simulink model "Hector_Simulation"  (R2023b)
settings: Solver=daessc  StartTime=0.0  StopTime=8  FixedStep=0.001  MaxStep=1e-3  RelTol=1e-2
model workspace (MATLAB code in the model file):
  | %% World Plane
  | plane_x = 20;
  | plane_y = 2;
  | plane_z = 0.05;
  | 
  | %% motor
  | %A1
  | motor_com = [0, -0.02,0];
  | motor_com_mirror = [0, 0.02,0];
  | 
  | motor_I = [0.00048,0.00071,0.00048];
  | motor_mass = 0.605;
  | 
  | %% Body
  | % Inertial
  | body_com_x = 0.0;
  | body_com_y = 0.0;
  | body_com_z = -0.0;
  | body_mass = 5.75;
  | body_ixx = 44350*1e-6;
  | body_ixy = 0.0;
  | body_ixz = 0.0;
  | body_iyy = 53149*1e-6;
  | body_iyz = 0.0;
  | body_izz = 21390*1e-6;
  | 
  | %% Hip 1
  | % joint
  | hip1_offset_x =0.0;
  | hip1_offset_y = 0.047;
  | hip1_offset_z = 0.1265;
  | % hip1_max = 15;
  | % hip1_min = -15;
  | hip1_velocity_max = 21;
  | hip1_torque_max = 33.5;
  | % Inertial
  | hip1_com_x = 0.0268;
  | hip1_com_y = -0.00315;
  | hip1_com_z = -0.0272;
  | hip1_mass = 0.173;
  | hip1_ixx = 0.00022;
  | hip1_ixy = 0.0;
  | hip1_ixz = 0.0;
  | hip1_iyy = 0.00024;
  | hip1_iyz = 0.0;
  | hip1_izz = 0.00016;
  | 
  | %% Hip 2
  | % joint
  | hip2_offset_x =0.053;
  | hip2_offset_y = 0.0185;
  | hip2_offset_z = 0.071;
  | % hip2_max = 15;
  | % hip2_min = -15;
  | hip2_velocity_max = 21;
  | hip2_torque_max = 33.5;
  | % Inertial
  | hip2_com_x = -0.0308;
  | hip2_com_y = -0.00942;
  | hip2_com_z = 0.0;
  | hip2_mass = 0.0722;
  | hip2_ixx = 0.0000422;
  | hip2_ixy = 0.0;
  | hip2_ixz = 0.0;
  | hip2_iyy = 0.000120;
  | hip2_iyz = 0.0;
  | hip2_izz = 0.0000708;
  | 
  | %% Thigh
  | % joint
  | thigh_offset_x =-0.06;
  | thigh_offset_y = 0.004;
  | thigh_offset_z = 0.0;
  | % thigh_max = 130;
  | % thigh_min = -45;
  | thigh_velocity_max = 21;
  | thigh_torque_max = 33.5;
  | % Inertial
  | thigh_com_x = -0.00143;
  | thigh_com_y = -0.02106;
  | thigh_com_z = -0.06115;
  | thigh_mass = 0.397;
  | thigh_ixx = 0.00197;
  | thigh_ixy = 0.0;
  | thigh_ixz = 0.0;
  | thigh_iyy = 0.00218;
  | thigh_iyz = 0.0;
  | thigh_izz = 0.00033;
  | 
  | ankle_motor_offset_x = 0;
  | ankle_motor_offset_y = 0.039;
  | ankle_motor_offset_z = 0;
  | 
  | knee_motor_offset_x = 0;
  | knee_motor_offset_y = 0.039;
  | knee_motor_offset_z = -0.095;
  | 
  | %% Calf
  | % joint
  | calf_offset_x = 0.0;
  | calf_offset_y = 0.003;
  | calf_offset_z = -0.22;
  | % calf_max = 0;
  | % calf_min = -135;
  | % knee_max = 0;
  | % knee_min = -160;
  | calf_velocity_max = 14*1.5;
  | calf_torque_max = 51;
  | % Inertial
  | calf_com_x = 0.00165;
  | calf_com_y = -0.01117;
  | calf_com_z = -0.06438;
  | calf_mass = 0.136;
  | calf_ixx = 0.00071;
  | calf_ixy = 0.0;
  | calf_ixz = 0.0;
  | calf_iyy = 0.00072;
  | calf_iyz = 0.0;
  | calf_izz = 0.00002;
  | 
  | %% Toe
  | % joint
  | toe_offset_x = 0.0;
  | toe_offset_y = 0.011;
  | toe_offset_z = -0.22;
  | % toe_max = 60;
  | % toe_min = -60;
  | toe_velocity_max = 21;
  | toe_torque_max = 33.5;
  | % Inertial
  | toe_com_x = 0.00239;
  | toe_com_y = 0.00002;
  | toe_com_z = -0.02261;
  | toe_mass = 0.08425;
  | toe_ixx = 0.00001;
  | toe_ixy = 0.0;
  | toe_ixz = 0.0;
  | toe_iyy = 0.00011;
  | toe_iyz = 0.0;
  | toe_izz = 0.00011;
  | %% Contact
  | contact_front = 0.091;
  | contact_rear = -0.061;
  | contact_right = 0.026;
  | contact_left = 0.01;
  | contact_z = 0.039;
  | 
  | %%
  | %dorito
  | dorito_offset_x = 0;
  | dorito_offset_y = 0.012;
  | dorito_offset_z = 0;
  | 
  | dorito_lower_connection = [0.034 0 -0.044];
  | dorito_upper_connection = [0.034 0 0.021];
  | 
  | linkage_mass = 0.051;
  | linkage_com = [0 0 -0.11];
  | linkage_I = [0.00001 0.00002 0.00002];
  | %% Arms
  | shoulder_com_x = 0;
  | shoulder_com_y = 0;
  | shoulder_com_z = 0;
  | shoulder_mass = 0.835;
  | % shoulder_mass = 0.05;
  | shoulder_ixx = 920*1e-6;
  | shoulder_ixy = 0.0;
  | shoulder_ixz = 0.0;
  | shoulder_iyy = 270*1e-6;
  | shoulder_iyz = 0.0;
  | shoulder_izz = 499*1e-6;
  | 
  | upperarm_com_x = 0;
  | upperarm_com_y = 0;
  | upperarm_com_z = 0;
  | upperarm_mass = 1.35;
  | % upperarm_mass = 0.05;
  | upperarm_ixx = 1200*1e-6;
  | upperarm_ixy = 0.0;
  | upperarm_ixz = 0.0;
  | upperarm_iyy = 1170*1e-6;
  | upperarm_iyz = 0.0;
  | upperarm_izz = 729*1e-6;
  | 
  | forearm_com_x = 0;
  | forearm_com_y = 0;
  | forearm_com_z = -0.10;
  | forearm_mass = 0.53;
  | % forearm_mass = 0.03;
  | forearm_ixx = 427*1e-6;
  | forearm_ixy = 0.0;
  | forearm_ixz = 0.0;
  | forearm_iyy = 466*1e-6;
  | forearm_iyz = 0.0;
  | forearm_izz = 72*1e-6;
values from neighbouring files (symbols this model uses):
  body_v0 = [0 0 0]    [Initiate_Simulation.m]
  body_z0 = 0.55    [Initiate_Simulation.m]
  dt_MPC = gaitcycle/10    (= 0.04)    [Initiate_Simulation.m]
  map = rot90(z_heights) > 0    [Occupancy_Map.m]
  N = 5000    [Initiate_Simulation.m]
  q_goal = [4; 0; body_z0]    [Initiate_Simulation.m]    (also in artificialPotential.m = reshape(u(3:4), 2, 1); main.m = [20; 20])
  shoulderx_max = 90    [Initiate_Simulation.m]
  shoulderx_min = -15    [Initiate_Simulation.m]
  shoulderx_q0 = 0    [Initiate_Simulation.m]
undefined symbols (not defined in the file or in its folder): AssignMPCStage, sigbuilder_block, X, Y, Z
libraries: sm_lib x169, nesl_utility x95, dspindex x1, simulink x1
(part 6 of 7)

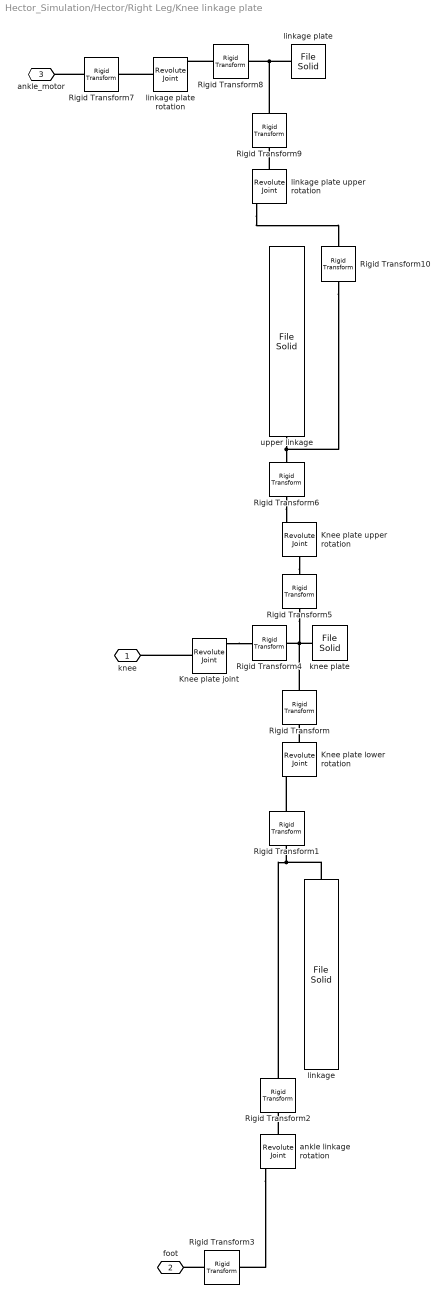
== system Hector_Simulation/Hector/Right Leg/Knee linkage plate ==
  Knee plate joint : sm_lib/Joints/Revolute Joint  JointMode=Normal  SenseConstraintForce=off  SenseConstraintForceX=off  SenseConstraintForceY=off  SenseConstraintForceZ=off  SenseConstraintTorque=off  SenseConstraintTorqueX=off  SenseConstraintTorqueY=off  SenseConstraintTorqueZ=off  SenseTotalForce=off  SenseTotalForceX=off  SenseTotalForceY=off  SenseTotalForceZ=off  SenseTotalTorque=off  SenseTotalTorqueX=off  SenseTotalTorqueY=off  SenseTotalTorqueZ=off  CompositeWrenchDir=FollowerOnBase  CompositeWrenchFrame=BaseFrame  EquilibriumPosition=0  EquilibriumPositionUnits=deg  SpringStiffness=0  SpringStiffnessUnits=N*m/deg  DampingCoefficient=joint_damping  DampingCoefficientUnits=N*m/(rad/s)  TorqueActuationMode=NoTorque  MotionActuationMode=ComputedMotion  SensePosition=on  SenseVelocity=on  SenseAcceleration=off  SenseTorqueForce=off  SenseLowerLimitTorqueForce=off  SenseUpperLimitTorqueForce=off  LowerLimitSpecify=off  LowerLimitBound=knee_min  LowerLimitBoundUnits=deg  LowerLimitStiffness=limit_stiffness  LowerLimitStiffnessUnits=N*m/deg  LowerLimitDamping=limit_damping  LowerLimitDampingUnits=N*m/(deg/s)  LowerLimitTransitionRegionWidth=0.1  LowerLimitTransitionRegionWidthUnits=deg  UpperLimitSpecify=off  UpperLimitBound=knee_max  UpperLimitBoundUnits=deg  UpperLimitStiffness=limit_stiffness  UpperLimitStiffnessUnits=N*m/deg  UpperLimitDamping=limit_damping  UpperLimitDampingUnits=N*m/(deg/s)  UpperLimitTransitionRegionWidth=0.1  UpperLimitTransitionRegionWidthUnits=deg  PositionTargetSpecify=off  PositionTargetPriority=High  PositionTargetValue=calf_q0  PositionTargetValueUnits=deg  VelocityTargetSpecify=off  VelocityTargetPriority=High  VelocityTargetValue=0  VelocityTargetValueUnits=deg/s
  Knee plate lower rotation : sm_lib/Joints/Revolute Joint  JointMode=Normal  SenseConstraintForce=off  SenseConstraintForceX=off  SenseConstraintForceY=off  SenseConstraintForceZ=off  SenseConstraintTorque=off  SenseConstraintTorqueX=off  SenseConstraintTorqueY=off  SenseConstraintTorqueZ=off  SenseTotalForce=off  SenseTotalForceX=off  SenseTotalForceY=off  SenseTotalForceZ=off  SenseTotalTorque=off  SenseTotalTorqueX=off  SenseTotalTorqueY=off  SenseTotalTorqueZ=off  CompositeWrenchDir=FollowerOnBase  CompositeWrenchFrame=BaseFrame  EquilibriumPosition=0  EquilibriumPositionUnits=deg  SpringStiffness=0  SpringStiffnessUnits=N*m/deg  DampingCoefficient=joint_damping  DampingCoefficientUnits=N*m/(rad/s)  TorqueActuationMode=NoTorque  MotionActuationMode=ComputedMotion  SensePosition=on  SenseVelocity=on  SenseAcceleration=off  SenseTorqueForce=off  SenseLowerLimitTorqueForce=off  SenseUpperLimitTorqueForce=off  LowerLimitSpecify=off  LowerLimitBound=knee_min  LowerLimitBoundUnits=deg  LowerLimitStiffness=limit_stiffness  LowerLimitStiffnessUnits=N*m/deg  LowerLimitDamping=limit_damping  LowerLimitDampingUnits=N*m/(deg/s)  LowerLimitTransitionRegionWidth=0.1  LowerLimitTransitionRegionWidthUnits=deg  UpperLimitSpecify=off  UpperLimitBound=knee_max  UpperLimitBoundUnits=deg  UpperLimitStiffness=limit_stiffness  UpperLimitStiffnessUnits=N*m/deg  UpperLimitDamping=limit_damping  UpperLimitDampingUnits=N*m/(deg/s)  UpperLimitTransitionRegionWidth=0.1  UpperLimitTransitionRegionWidthUnits=deg  PositionTargetSpecify=off  PositionTargetPriority=High  PositionTargetValue=calf_q0  PositionTargetValueUnits=deg  VelocityTargetSpecify=off  VelocityTargetPriority=High  VelocityTargetValue=0  VelocityTargetValueUnits=deg/s
  Knee plate upper rotation : sm_lib/Joints/Revolute Joint  JointMode=Normal  SenseConstraintForce=off  SenseConstraintForceX=off  SenseConstraintForceY=off  SenseConstraintForceZ=off  SenseConstraintTorque=off  SenseConstraintTorqueX=off  SenseConstraintTorqueY=off  SenseConstraintTorqueZ=off  SenseTotalForce=off  SenseTotalForceX=off  SenseTotalForceY=off  SenseTotalForceZ=off  SenseTotalTorque=off  SenseTotalTorqueX=off  SenseTotalTorqueY=off  SenseTotalTorqueZ=off  CompositeWrenchDir=FollowerOnBase  CompositeWrenchFrame=BaseFrame  EquilibriumPosition=0  EquilibriumPositionUnits=deg  SpringStiffness=0  SpringStiffnessUnits=N*m/deg  DampingCoefficient=joint_damping  DampingCoefficientUnits=N*m/(rad/s)  TorqueActuationMode=NoTorque  MotionActuationMode=ComputedMotion  SensePosition=on  SenseVelocity=on  SenseAcceleration=off  SenseTorqueForce=off  SenseLowerLimitTorqueForce=off  SenseUpperLimitTorqueForce=off  LowerLimitSpecify=off  LowerLimitBound=knee_min  LowerLimitBoundUnits=deg  LowerLimitStiffness=limit_stiffness  LowerLimitStiffnessUnits=N*m/deg  LowerLimitDamping=limit_damping  LowerLimitDampingUnits=N*m/(deg/s)  LowerLimitTransitionRegionWidth=0.1  LowerLimitTransitionRegionWidthUnits=deg  UpperLimitSpecify=off  UpperLimitBound=knee_max  UpperLimitBoundUnits=deg  UpperLimitStiffness=limit_stiffness  UpperLimitStiffnessUnits=N*m/deg  UpperLimitDamping=limit_damping  UpperLimitDampingUnits=N*m/(deg/s)  UpperLimitTransitionRegionWidth=0.1  UpperLimitTransitionRegionWidthUnits=deg  PositionTargetSpecify=off  PositionTargetPriority=High  PositionTargetValue=calf_q0  PositionTargetValueUnits=deg  VelocityTargetSpecify=off  VelocityTargetPriority=High  VelocityTargetValue=0  VelocityTargetValueUnits=deg/s
  Rigid Transform : sm_lib/Frames and Transforms/Rigid Transform  TranslationMethod=Cartesian  TranslationStandardOffset=0  TranslationStandardOffsetUnits=m  TranslationStandardAxis=+Z  TranslationCartesianOffset=dorito_lower_connection  TranslationCartesianOffsetUnits=m  TranslationROffset=0  TranslationROffsetUnits=m  TranslationZOffset=0  TranslationZOffsetUnits=m  TranslationThetaOffset=0  TranslationThetaOffsetUnits=deg  RotationMethod=StandardAxis  RotationAngleUnits=deg  RotationStandardAxis=+X  RotationAngle=90  RotationArbitraryAxis=[0 0 1]  FollAlignAxisA=+X  BaseAlignAxisA=+Y  FollAlignAxisB=+Y  BaseAlignAxisB=+Z  RotationSequenceAxes=FollowerAxes  RotationSequence=XYX  RotationSequenceAngles=[0 0 0]  RotationSequenceAnglesUnits=deg  RotationMatrix=[1 0 0; 0 1 0; 0 0 1]  Quaternion=[1 0 0 0]
  Rigid Transform1 : sm_lib/Frames and Transforms/Rigid Transform  TranslationMethod=None  TranslationStandardOffset=0  TranslationStandardOffsetUnits=m  TranslationStandardAxis=+Z  TranslationCartesianOffset=dorito_lower_connection  TranslationCartesianOffsetUnits=m  TranslationROffset=0  TranslationROffsetUnits=m  TranslationZOffset=0  TranslationZOffsetUnits=m  TranslationThetaOffset=0  TranslationThetaOffsetUnits=deg  RotationMethod=RotationSequence  RotationAngleUnits=deg  RotationStandardAxis=+X  RotationAngle=90  RotationArbitraryAxis=[0 0 1]  FollAlignAxisA=+X  BaseAlignAxisA=+Y  FollAlignAxisB=+Y  BaseAlignAxisB=+Z  RotationSequenceAxes=FollowerAxes  RotationSequence=XYZ  RotationSequenceAngles=[0 90 90]  RotationSequenceAnglesUnits=deg  RotationMatrix=[1 0 0; 0 1 0; 0 0 1]  Quaternion=[1 0 0 0]
  Rigid Transform10 : sm_lib/Frames and Transforms/Rigid Transform  TranslationMethod=Cartesian  TranslationStandardOffset=0  TranslationStandardOffsetUnits=m  TranslationStandardAxis=+Z  TranslationCartesianOffset=[0 0 -0.22]  TranslationCartesianOffsetUnits=m  TranslationROffset=0  TranslationROffsetUnits=m  TranslationZOffset=0  TranslationZOffsetUnits=m  TranslationThetaOffset=0  TranslationThetaOffsetUnits=deg  RotationMethod=StandardAxis  RotationAngleUnits=deg  RotationStandardAxis=-X  RotationAngle=90  RotationArbitraryAxis=[0 0 1]  FollAlignAxisA=+X  BaseAlignAxisA=+Y  FollAlignAxisB=+Y  BaseAlignAxisB=+Z  RotationSequenceAxes=FollowerAxes  RotationSequence=XYZ  RotationSequenceAngles=[0 90 90]  RotationSequenceAnglesUnits=deg  RotationMatrix=[1 0 0; 0 1 0; 0 0 1]  Quaternion=[1 0 0 0]
  Rigid Transform2 : sm_lib/Frames and Transforms/Rigid Transform  TranslationMethod=Cartesian  TranslationStandardOffset=0  TranslationStandardOffsetUnits=m  TranslationStandardAxis=+Z  TranslationCartesianOffset=[0 0 -0.22]  TranslationCartesianOffsetUnits=m  TranslationROffset=0  TranslationROffsetUnits=m  TranslationZOffset=0  TranslationZOffsetUnits=m  TranslationThetaOffset=0  TranslationThetaOffsetUnits=deg  RotationMethod=RotationSequence  RotationAngleUnits=deg  RotationStandardAxis=+X  RotationAngle=90  RotationArbitraryAxis=[0 0 1]  FollAlignAxisA=+X  BaseAlignAxisA=+Y  FollAlignAxisB=+Y  BaseAlignAxisB=+Z  RotationSequenceAxes=FollowerAxes  RotationSequence=XYZ  RotationSequenceAngles=[-90 0 0]  RotationSequenceAnglesUnits=deg  RotationMatrix=[1 0 0; 0 1 0; 0 0 1]  Quaternion=[1 0 0 0]
  Rigid Transform3 : sm_lib/Frames and Transforms/Rigid Transform  TranslationMethod=Cartesian  TranslationStandardOffset=0  TranslationStandardOffsetUnits=m  TranslationStandardAxis=+Z  TranslationCartesianOffset=[0.0475 -0.0275 0.001 ]  TranslationCartesianOffsetUnits=m  TranslationROffset=0  TranslationROffsetUnits=m  TranslationZOffset=0  TranslationZOffsetUnits=m  TranslationThetaOffset=0  TranslationThetaOffsetUnits=deg  RotationMethod=StandardAxis  RotationAngleUnits=deg  RotationStandardAxis=+X  RotationAngle=90  RotationArbitraryAxis=[0 0 1]  FollAlignAxisA=+X  BaseAlignAxisA=+Y  FollAlignAxisB=+Y  BaseAlignAxisB=+Z  RotationSequenceAxes=FollowerAxes  RotationSequence=XYZ  RotationSequenceAngles=[90 0 180]  RotationSequenceAnglesUnits=deg  RotationMatrix=[1 0 0; 0 1 0; 0 0 1]  Quaternion=[1 0 0 0]
  Rigid Transform4 : sm_lib/Frames and Transforms/Rigid Transform  TranslationMethod=Cartesian  TranslationStandardOffset=0  TranslationStandardOffsetUnits=m  TranslationStandardAxis=+Z  TranslationCartesianOffset=[dorito_offset_x -dorito_offset_y dorito_offset_z]  TranslationCartesianOffsetUnits=m  TranslationROffset=0  TranslationROffsetUnits=m  TranslationZOffset=0  TranslationZOffsetUnits=m  TranslationThetaOffset=0  TranslationThetaOffsetUnits=deg  RotationMethod=RotationSequence  RotationAngleUnits=deg  RotationStandardAxis=+Z  RotationAngle=90  RotationArbitraryAxis=[0 0 1]  FollAlignAxisA=+X  BaseAlignAxisA=+Y  FollAlignAxisB=+Y  BaseAlignAxisB=+Z  RotationSequenceAxes=FollowerAxes  RotationSequence=XYZ  RotationSequenceAngles=[90 0 180]  RotationSequenceAnglesUnits=deg  RotationMatrix=[1 0 0; 0 1 0; 0 0 1]  Quaternion=[1 0 0 0]
  Rigid Transform5 : sm_lib/Frames and Transforms/Rigid Transform  TranslationMethod=Cartesian  TranslationStandardOffset=0  TranslationStandardOffsetUnits=m  TranslationStandardAxis=+Z  TranslationCartesianOffset=[dorito_upper_connection(1), dorito_upper_connection(2), dorito_upper_connection(3)]  TranslationCartesianOffsetUnits=m  TranslationROffset=0  TranslationROffsetUnits=m  TranslationZOffset=0  TranslationZOffsetUnits=m  TranslationThetaOffset=0  TranslationThetaOffsetUnits=deg  RotationMethod=StandardAxis  RotationAngleUnits=deg  RotationStandardAxis=+X  RotationAngle=90  RotationArbitraryAxis=[0 0 1]  FollAlignAxisA=+X  BaseAlignAxisA=+Y  FollAlignAxisB=+Y  BaseAlignAxisB=+Z  RotationSequenceAxes=FollowerAxes  RotationSequence=XYX  RotationSequenceAngles=[0 0 0]  RotationSequenceAnglesUnits=deg  RotationMatrix=[1 0 0; 0 1 0; 0 0 1]  Quaternion=[1 0 0 0]
  Rigid Transform6 : sm_lib/Frames and Transforms/Rigid Transform  TranslationMethod=None  TranslationStandardOffset=0  TranslationStandardOffsetUnits=m  TranslationStandardAxis=+Z  TranslationCartesianOffset=dorito_lower_connection  TranslationCartesianOffsetUnits=m  TranslationROffset=0  TranslationROffsetUnits=m  TranslationZOffset=0  TranslationZOffsetUnits=m  TranslationThetaOffset=0  TranslationThetaOffsetUnits=deg  RotationMethod=RotationSequence  RotationAngleUnits=deg  RotationStandardAxis=+X  RotationAngle=90  RotationArbitraryAxis=[0 0 1]  FollAlignAxisA=+X  BaseAlignAxisA=+Y  FollAlignAxisB=+Y  BaseAlignAxisB=+Z  RotationSequenceAxes=FollowerAxes  RotationSequence=XYZ  RotationSequenceAngles=[0 90 90]  RotationSequenceAnglesUnits=deg  RotationMatrix=[1 0 0; 0 1 0; 0 0 1]  Quaternion=[1 0 0 0]
  Rigid Transform7 : sm_lib/Frames and Transforms/Rigid Transform  TranslationMethod=Cartesian  TranslationStandardOffset=0  TranslationStandardOffsetUnits=m  TranslationStandardAxis=+Z  TranslationCartesianOffset=[0 -0.014 0]  TranslationCartesianOffsetUnits=m  TranslationROffset=0  TranslationROffsetUnits=m  TranslationZOffset=0  TranslationZOffsetUnits=m  TranslationThetaOffset=0  TranslationThetaOffsetUnits=deg  RotationMethod=StandardAxis  RotationAngleUnits=deg  RotationStandardAxis=+X  RotationAngle=90  RotationArbitraryAxis=[0 0 1]  FollAlignAxisA=+X  BaseAlignAxisA=+Y  FollAlignAxisB=+Y  BaseAlignAxisB=+Z  RotationSequenceAxes=FollowerAxes  RotationSequence=XYX  RotationSequenceAngles=[0 0 0]  RotationSequenceAnglesUnits=deg  RotationMatrix=[1 0 0; 0 1 0; 0 0 1]  Quaternion=[1 0 0 0]
  Rigid Transform8 : sm_lib/Frames and Transforms/Rigid Transform  TranslationMethod=Cartesian  TranslationStandardOffset=0  TranslationStandardOffsetUnits=m  TranslationStandardAxis=+Z  TranslationCartesianOffset=[0 0.00001 0]  TranslationCartesianOffsetUnits=m  TranslationROffset=0  TranslationROffsetUnits=m  TranslationZOffset=0  TranslationZOffsetUnits=m  TranslationThetaOffset=0  TranslationThetaOffsetUnits=deg  RotationMethod=RotationSequence  RotationAngleUnits=deg  RotationStandardAxis=+X  RotationAngle=90  RotationArbitraryAxis=[0 0 1]  FollAlignAxisA=+X  BaseAlignAxisA=+Y  FollAlignAxisB=+Y  BaseAlignAxisB=+Z  RotationSequenceAxes=BaseAxes  RotationSequence=XYX  RotationSequenceAngles=[0 90 90]  RotationSequenceAnglesUnits=deg  RotationMatrix=[1 0 0; 0 1 0; 0 0 1]  Quaternion=[1 0 0 0]
  Rigid Transform9 : sm_lib/Frames and Transforms/Rigid Transform  TranslationMethod=Cartesian  TranslationStandardOffset=0  TranslationStandardOffsetUnits=m  TranslationStandardAxis=+Z  TranslationCartesianOffset=[0.038 0.013 -0.01]  TranslationCartesianOffsetUnits=m  TranslationROffset=0  TranslationROffsetUnits=m  TranslationZOffset=0  TranslationZOffsetUnits=m  TranslationThetaOffset=0  TranslationThetaOffsetUnits=deg  RotationMethod=RotationSequence  RotationAngleUnits=deg  RotationStandardAxis=+X  RotationAngle=90  RotationArbitraryAxis=[0 0 1]  FollAlignAxisA=+X  BaseAlignAxisA=+Y  FollAlignAxisB=+Y  BaseAlignAxisB=+Z  RotationSequenceAxes=BaseAxes  RotationSequence=XYX  RotationSequenceAngles=[90 0 0]  RotationSequenceAnglesUnits=deg  RotationMatrix=[1 0 0; 0 1 0; 0 0 1]  Quaternion=[1 0 0 0]
  ankle linkage rotation : sm_lib/Joints/Revolute Joint  JointMode=Normal  SenseConstraintForce=off  SenseConstraintForceX=off  SenseConstraintForceY=off  SenseConstraintForceZ=off  SenseConstraintTorque=off  SenseConstraintTorqueX=off  SenseConstraintTorqueY=off  SenseConstraintTorqueZ=off  SenseTotalForce=off  SenseTotalForceX=off  SenseTotalForceY=off  SenseTotalForceZ=off  SenseTotalTorque=off  SenseTotalTorqueX=off  SenseTotalTorqueY=off  SenseTotalTorqueZ=off  CompositeWrenchDir=FollowerOnBase  CompositeWrenchFrame=BaseFrame  EquilibriumPosition=0  EquilibriumPositionUnits=deg  SpringStiffness=0  SpringStiffnessUnits=N*m/deg  DampingCoefficient=joint_damping  DampingCoefficientUnits=N*m/(rad/s)  TorqueActuationMode=NoTorque  MotionActuationMode=ComputedMotion  SensePosition=on  SenseVelocity=on  SenseAcceleration=off  SenseTorqueForce=off  SenseLowerLimitTorqueForce=off  SenseUpperLimitTorqueForce=off  LowerLimitSpecify=off  LowerLimitBound=knee_min  LowerLimitBoundUnits=deg  LowerLimitStiffness=limit_stiffness  LowerLimitStiffnessUnits=N*m/deg  LowerLimitDamping=limit_damping  LowerLimitDampingUnits=N*m/(deg/s)  LowerLimitTransitionRegionWidth=0.1  LowerLimitTransitionRegionWidthUnits=deg  UpperLimitSpecify=off  UpperLimitBound=knee_max  UpperLimitBoundUnits=deg  UpperLimitStiffness=limit_stiffness  UpperLimitStiffnessUnits=N*m/deg  UpperLimitDamping=limit_damping  UpperLimitDampingUnits=N*m/(deg/s)  UpperLimitTransitionRegionWidth=0.1  UpperLimitTransitionRegionWidthUnits=deg  PositionTargetSpecify=off  PositionTargetPriority=High  PositionTargetValue=calf_q0  PositionTargetValueUnits=deg  VelocityTargetSpecify=off  VelocityTargetPriority=High  VelocityTargetValue=0  VelocityTargetValueUnits=deg/s
  knee plate : sm_lib/Body Elements/File Solid  ExtGeomFileName=STL files\Dorito.stl  UnitType=Custom  ExtGeomFileUnits=m  StepReaderType=HEX  ExportConvexHullGeometry=off  InertiaType=PointMass  Mass=0.03  MassUnits=kg  CenterOfMass=[calf_com_x -calf_com_y calf_com_z]  CenterOfMassUnits=m  MomentsOfInertia=[calf_ixx calf_iyy calf_izz]  MomentsOfInertiaUnits=kg*m^2  ProductsOfInertia=[0 0 0]  ProductsOfInertiaUnits=kg*m^2  BasedOnType=Density  Density=1000  DensityUnits=kg/m^3  DoExposeReferenceFrame=on  SerializedFrames=<Frames/>  GraphicType=FromGeometry  MarkerShape=Sphere  MarkerSize=10  GraphicVisPropType=AdvancedVisualProperties  GraphicDiffuseColor=[0.9 0.9 0.9]  GraphicSpecularColor=[0.7 0.7 0.7 1.0]  GraphicAmbientColor=[0.35 0.35 0.35 1.0]  GraphicEmissiveColor=[0.0 0.0 0.0 1.0]  GraphicShininess=5  GraphicOpacity=1.0
  linkage : sm_lib/Body Elements/File Solid  ExtGeomFileName=STL files\linkage.stl  UnitType=Custom  ExtGeomFileUnits=m  StepReaderType=HEX  ExportConvexHullGeometry=off  InertiaType=Custom  Mass=linkage_mass  MassUnits=kg  CenterOfMass=linkage_com  CenterOfMassUnits=m  MomentsOfInertia=linkage_I  MomentsOfInertiaUnits=kg*m^2  ProductsOfInertia=[0 0 0]  ProductsOfInertiaUnits=kg*m^2  BasedOnType=Density  Density=1000  DensityUnits=kg/m^3  DoExposeReferenceFrame=on  SerializedFrames=<Frames/>  GraphicType=FromGeometry  MarkerShape=Sphere  MarkerSize=10  GraphicVisPropType=AdvancedVisualProperties  GraphicDiffuseColor=[0.9 0.9 0.9]  GraphicSpecularColor=[0.7 0.7 0.7 1.0]  GraphicAmbientColor=[0.35 0.35 0.35 1.0]  GraphicEmissiveColor=[0.0 0.0 0.0 1.0]  GraphicShininess=5  GraphicOpacity=1.0
  linkage plate : sm_lib/Body Elements/File Solid  ExtGeomFileName=STL files\R_linkage_plate.stl  UnitType=Custom  ExtGeomFileUnits=m  StepReaderType=HEX  ExportConvexHullGeometry=off  InertiaType=PointMass  Mass=0.03  MassUnits=kg  CenterOfMass=[calf_com_x -calf_com_y calf_com_z]  CenterOfMassUnits=m  MomentsOfInertia=[calf_ixx calf_iyy calf_izz]  MomentsOfInertiaUnits=kg*m^2  ProductsOfInertia=[0 0 0]  ProductsOfInertiaUnits=kg*m^2  BasedOnType=Density  Density=1000  DensityUnits=kg/m^3  DoExposeReferenceFrame=on  SerializedFrames=<Frames/>  GraphicType=FromGeometry  MarkerShape=Sphere  MarkerSize=10  GraphicVisPropType=AdvancedVisualProperties  GraphicDiffuseColor=[0.9 0.9 0.9]  GraphicSpecularColor=[0.7 0.7 0.7 1.0]  GraphicAmbientColor=[0.35 0.35 0.35 1.0]  GraphicEmissiveColor=[0.0 0.0 0.0 1.0]  GraphicShininess=5  GraphicOpacity=1.0
  linkage plate rotation : sm_lib/Joints/Revolute Joint  JointMode=Normal  SenseConstraintForce=off  SenseConstraintForceX=off  SenseConstraintForceY=off  SenseConstraintForceZ=off  SenseConstraintTorque=off  SenseConstraintTorqueX=off  SenseConstraintTorqueY=off  SenseConstraintTorqueZ=off  SenseTotalForce=off  SenseTotalForceX=off  SenseTotalForceY=off  SenseTotalForceZ=off  SenseTotalTorque=off  SenseTotalTorqueX=off  SenseTotalTorqueY=off  SenseTotalTorqueZ=off  CompositeWrenchDir=FollowerOnBase  CompositeWrenchFrame=BaseFrame  EquilibriumPosition=0  EquilibriumPositionUnits=deg  SpringStiffness=0  SpringStiffnessUnits=N*m/deg  DampingCoefficient=joint_damping  DampingCoefficientUnits=N*m/(rad/s)  TorqueActuationMode=NoTorque  MotionActuationMode=ComputedMotion  SensePosition=on  SenseVelocity=on  SenseAcceleration=off  SenseTorqueForce=off  SenseLowerLimitTorqueForce=off  SenseUpperLimitTorqueForce=off  LowerLimitSpecify=off  LowerLimitBound=knee_min  LowerLimitBoundUnits=deg  LowerLimitStiffness=limit_stiffness  LowerLimitStiffnessUnits=N*m/deg  LowerLimitDamping=limit_damping  LowerLimitDampingUnits=N*m/(deg/s)  LowerLimitTransitionRegionWidth=0.1  LowerLimitTransitionRegionWidthUnits=deg  UpperLimitSpecify=off  UpperLimitBound=knee_max  UpperLimitBoundUnits=deg  UpperLimitStiffness=limit_stiffness  UpperLimitStiffnessUnits=N*m/deg  UpperLimitDamping=limit_damping  UpperLimitDampingUnits=N*m/(deg/s)  UpperLimitTransitionRegionWidth=0.1  UpperLimitTransitionRegionWidthUnits=deg  PositionTargetSpecify=off  PositionTargetPriority=High  PositionTargetValue=calf_q0  PositionTargetValueUnits=deg  VelocityTargetSpecify=off  VelocityTargetPriority=High  VelocityTargetValue=0  VelocityTargetValueUnits=deg/s
  linkage plate upper rotation : sm_lib/Joints/Revolute Joint  JointMode=Normal  SenseConstraintForce=off  SenseConstraintForceX=off  SenseConstraintForceY=off  SenseConstraintForceZ=off  SenseConstraintTorque=off  SenseConstraintTorqueX=off  SenseConstraintTorqueY=off  SenseConstraintTorqueZ=off  SenseTotalForce=off  SenseTotalForceX=off  SenseTotalForceY=off  SenseTotalForceZ=off  SenseTotalTorque=off  SenseTotalTorqueX=off  SenseTotalTorqueY=off  SenseTotalTorqueZ=off  CompositeWrenchDir=FollowerOnBase  CompositeWrenchFrame=BaseFrame  EquilibriumPosition=0  EquilibriumPositionUnits=deg  SpringStiffness=0  SpringStiffnessUnits=N*m/deg  DampingCoefficient=joint_damping  DampingCoefficientUnits=N*m/(rad/s)  TorqueActuationMode=NoTorque  MotionActuationMode=ComputedMotion  SensePosition=on  SenseVelocity=on  SenseAcceleration=off  SenseTorqueForce=off  SenseLowerLimitTorqueForce=off  SenseUpperLimitTorqueForce=off  LowerLimitSpecify=off  LowerLimitBound=knee_min  LowerLimitBoundUnits=deg  LowerLimitStiffness=limit_stiffness  LowerLimitStiffnessUnits=N*m/deg  LowerLimitDamping=limit_damping  LowerLimitDampingUnits=N*m/(deg/s)  LowerLimitTransitionRegionWidth=0.1  LowerLimitTransitionRegionWidthUnits=deg  UpperLimitSpecify=off  UpperLimitBound=knee_max  UpperLimitBoundUnits=deg  UpperLimitStiffness=limit_stiffness  UpperLimitStiffnessUnits=N*m/deg  UpperLimitDamping=limit_damping  UpperLimitDampingUnits=N*m/(deg/s)  UpperLimitTransitionRegionWidth=0.1  UpperLimitTransitionRegionWidthUnits=deg  PositionTargetSpecify=off  PositionTargetPriority=High  PositionTargetValue=calf_q0  PositionTargetValueUnits=deg  VelocityTargetSpecify=off  VelocityTargetPriority=High  VelocityTargetValue=0  VelocityTargetValueUnits=deg/s
  upper linkage : sm_lib/Body Elements/File Solid  ExtGeomFileName=STL files\linkage.stl  UnitType=Custom  ExtGeomFileUnits=m  StepReaderType=HEX  ExportConvexHullGeometry=off  InertiaType=Custom  Mass=linkage_mass  MassUnits=kg  CenterOfMass=linkage_com  CenterOfMassUnits=m  MomentsOfInertia=linkage_I  MomentsOfInertiaUnits=kg*m^2  ProductsOfInertia=[0 0 0]  ProductsOfInertiaUnits=kg*m^2  BasedOnType=Density  Density=1000  DensityUnits=kg/m^3  DoExposeReferenceFrame=on  SerializedFrames=<Frames/>  GraphicType=FromGeometry  MarkerShape=Sphere  MarkerSize=10  GraphicVisPropType=AdvancedVisualProperties  GraphicDiffuseColor=[0.9 0.9 0.9]  GraphicSpecularColor=[0.7 0.7 0.7 1.0]  GraphicAmbientColor=[0.35 0.35 0.35 1.0]  GraphicEmissiveColor=[0.0 0.0 0.0 1.0]  GraphicShininess=5  GraphicOpacity=1.0
  knee : PMIOPort  Side=Left
  foot : PMIOPort  Port=2  Side=Right
  ankle_motor : PMIOPort  Port=3  Side=Left
  connections:
  Rigid Transform/LConn1 -- knee plate/RConn1 -- Rigid Transform4/LConn1 -- Rigid Transform5/LConn1
  Knee plate joint/LConn1 -- knee/RConn1
  Knee plate joint/RConn1 -- Rigid Transform4/RConn1
  Knee plate lower rotation/LConn1 -- Rigid Transform/RConn1
  Rigid Transform1/LConn1 -- Knee plate lower rotation/RConn1
  linkage/RConn1 -- Rigid Transform1/RConn1 -- Rigid Transform2/LConn1
  ankle linkage rotation/LConn1 -- Rigid Transform2/RConn1
  Rigid Transform3/RConn1 -- foot/RConn1
  ankle linkage rotation/RConn1 -- Rigid Transform3/LConn1
  Knee plate upper rotation/LConn1 -- Rigid Transform5/RConn1
  Rigid Transform6/LConn1 -- Knee plate upper rotation/RConn1
  Rigid Transform6/RConn1 -- upper linkage/RConn1 -- Rigid Transform10/LConn1
  linkage plate rotation/LConn1 -- Rigid Transform7/RConn1
  Rigid Transform7/LConn1 -- ankle_motor/RConn1
  Rigid Transform8/LConn1 -- linkage plate rotation/RConn1
  linkage plate/RConn1 -- Rigid Transform9/RConn1 -- Rigid Transform8/RConn1
  linkage plate upper rotation/LConn1 -- Rigid Transform9/LConn1
  linkage plate upper rotation/RConn1 -- Rigid Transform10/RConn1

== system Hector_Simulation/Hector/Right Leg/Package Measurements 3D ==
  Fn : Inport
  Ff : Inport  Port=2
  ankle : Inport  Port=3
  knee : Inport  Port=4
  hip_pitch : Inport  Port=5
  hip_roll : Inport  Port=6
  hip_yaw : Inport  Port=7
  hip_location : Inport  Port=8
  foot_pos_vel : Inport  Port=9
  Bus Creator3 : BusCreator  Inputs=19
  Extract Measurements : Subsystem
  Extract Measurements1 : Subsystem
  Extract Measurements2 : Subsystem
  Extract Measurements3 : Subsystem
  Extract Measurements4 : Subsystem
  meas : Outport  VectorParamsAs1DForOutWhenUnconnected=off
  wires:
  Extract Measurements3/1(angle) -> Bus Creator3/12  "hip_roll_angle"
  Extract Measurements3/3(torque) -> Bus Creator3/14  "hip_roll_torque"
  hip_roll/1 -> Extract Measurements3/1(meas)
  Extract Measurements/3(torque) -> Bus Creator3/5  "ankle_torque"
  Extract Measurements/1(angle) -> Bus Creator3/3  "ankle_angle"
  ankle/1 -> Extract Measurements/1(meas)
  Bus Creator3/1 -> meas/1
  knee/1 -> Extract Measurements1/1(meas)
  Extract Measurements1/1(angle) -> Bus Creator3/6  "knee_angle"
  Extract Measurements1/3(torque) -> Bus Creator3/8  "knee_torque"
  hip_pitch/1 -> Extract Measurements2/1(meas)
  hip_yaw/1 -> Extract Measurements4/1(meas)
  Extract Measurements2/3(torque) -> Bus Creator3/11  "hip_pitch_torque"
  Extract Measurements4/1(angle) -> Bus Creator3/15  "hip_yaw_angle"
  Extract Measurements4/3(torque) -> Bus Creator3/17  "hip_yaw_torque"
  Ff/1 -> Bus Creator3/2  "friction_force"
  Fn/1 -> Bus Creator3/1  "normal_force"
  Extract Measurements/2(speed) -> Bus Creator3/4  "ankle_speed"
  Extract Measurements1/2(speed) -> Bus Creator3/7  "knee_speed"
  Extract Measurements2/1(angle) -> Bus Creator3/9  "hip_pitch_angle"
  Extract Measurements2/2(speed) -> Bus Creator3/10  "hip_pitch_speed"
  Extract Measurements3/2(speed) -> Bus Creator3/13  "hip_roll_speed"
  Extract Measurements4/2(speed) -> Bus Creator3/16  "hip_yaw_speed"
  hip_location/1 -> Bus Creator3/18  "hip_location_r"
  foot_pos_vel/1 -> Bus Creator3/19  "foot_pos_vel_r"

== system Hector_Simulation/Hector/Right Leg/Subsystem ==
  Bus Creator1 : BusCreator  Inputs=6
  PS-Simulink Converter{3..8} (6 alike) : nesl_utility/PS-Simulink Converter  PhysicalDomain=network_engine_domain  SubClassName=ps_output  LeftPortType=input  RightPortType=output  PseudoPeriodic=off  Frequencies=[]  VectorFormat=1-D array  Unit=inherit  AffineConversion=off
  Rigid Transform7 : sm_lib/Frames and Transforms/Rigid Transform  TranslationMethod=Cartesian  TranslationStandardOffset=0  TranslationStandardOffsetUnits=m  TranslationStandardAxis=+Z  TranslationCartesianOffset=[0 toe_com_y -contact_z]  TranslationCartesianOffsetUnits=m  TranslationROffset=0  TranslationROffsetUnits=m  TranslationZOffset=0  TranslationZOffsetUnits=m  TranslationThetaOffset=0  TranslationThetaOffsetUnits=deg  RotationMethod=None  RotationAngleUnits=deg  RotationStandardAxis=+Z  RotationAngle=0.0  RotationArbitraryAxis=[0 0 1]  FollAlignAxisA=+X  BaseAlignAxisA=+Y  FollAlignAxisB=+Y  BaseAlignAxisB=+Z  RotationSequenceAxes=FollowerAxes  RotationSequence=XYX  RotationSequenceAngles=[0 0 0]  RotationSequenceAnglesUnits=deg  RotationMatrix=[1 0 0; 0 1 0; 0 0 1]  Quaternion=[1 0 0 0]
  Scope : Scope
  Transform Sensor1 : sm_lib/Frames and Transforms/Transform Sensor  MeasurementFrame=World  RotationSequence=XYX  SenseAngle=off  SenseAxis=off  SenseQ=off  SenseR=off  SenseRotationSequence=off  SenseOmegaX=off  SenseOmegaY=off  SenseOmegaZ=off  SenseOmega=off  SenseQDot=off  SenseRDot=off  SenseRotationSequenceDot=off  SenseAlphaX=off  SenseAlphaY=off  SenseAlphaZ=off  SenseAlpha=off  SenseQDDot=off  SenseRDDot=off  SenseX=on  SenseY=on  SenseZ=on  SenseXYZ=off  SenseRad=off  SenseAzim=off  SenseDist=off  SenseInc=off  SenseXDot=on  SenseYDot=on  SenseZDot=on  SenseXYZDot=off  SenseRadDot=off  SenseAzimDot=off  SenseDistDot=off  SenseIncDot=off  SenseXDDot=off  SenseYDDot=off  SenseZDDot=off  SenseXYZDDot=off  SenseRadDDot=off  SenseAzimDDot=off  SenseDistDDot=off  SenseIncDDot=off
  World Frame1 : sm_lib/Frames and Transforms/World Frame
  R : PMIOPort  Side=Left
  foot_pos_vel : Outport
  wires:
  PS-Simulink Converter6/1 -> Bus Creator1/4  "vx"
  PS-Simulink Converter5/1 -> Scope/1, Bus Creator1/3  "z"
  PS-Simulink Converter7/1 -> Bus Creator1/5  "vy"
  PS-Simulink Converter4/1 -> Bus Creator1/2  "y"
  PS-Simulink Converter8/1 -> Bus Creator1/6  "vz"
  PS-Simulink Converter3/1 -> Bus Creator1/1  "x"
  Bus Creator1/1 -> foot_pos_vel/1
  connections:
  Rigid Transform7/RConn1 -- Transform Sensor1/RConn1
  R/RConn1 -- Rigid Transform7/LConn1
  Transform Sensor1/RConn7 -- PS-Simulink Converter8/LConn1
  Transform Sensor1/RConn6 -- PS-Simulink Converter7/LConn1
  PS-Simulink Converter4/LConn1 -- Transform Sensor1/RConn3
  Transform Sensor1/RConn4 -- PS-Simulink Converter5/LConn1
  Transform Sensor1/RConn5 -- PS-Simulink Converter6/LConn1
  Transform Sensor1/LConn1 -- World Frame1/RConn1
  PS-Simulink Converter3/LConn1 -- Transform Sensor1/RConn2

== system Hector_Simulation/Hector/Right Leg/Thigh ==
  Joint : Inport
  Hip Pitch Joint : Subsystem
      settings: PortSchema="{\"entries\":[{\"content\":{\"sides\":[{\"content\":{\"connectorIds\":[\"LConn1\",\"In1\"]},\"type\":\"ConnectorPlacement.EquallySpacedRectSide\",\"uuid\":\"fe1bafd1-c1a5-4148-b465-5de294b235b8\"},{\"content\":{\"connectorIds\":[\"RConn1\",\"Out1\"],\"side\":\"RIGHT\"},\"type\":\"ConnectorPlacement.EquallySpacedRectSide\",\"uuid\":\"cbba8e06-0841-4611-b08d-047237296da9\"},{\"content\":{\"connectorIds\":[],\"side\":\"TOP\"},\"type\":\"ConnectorPlacement.EquallySpacedRectSide\",\"uuid\":\"b5035594-e8f7-4741-b410-9cfafd0751b0\"}]},\"type\":\"ConnectorPlacement.EquallySpacedConnector\",\"uuid\":\"2233606c-74e6-45bf-8a73-f401921fd730\"}],\"packageUris\":[\"http://schema.mathworks.com/mf0/Connector/R2020b\"],\"version\":\"1.0\"}"
  Rigid Transform1 : sm_lib/Frames and Transforms/Rigid Transform  TranslationMethod=Cartesian  TranslationStandardOffset=0  TranslationStandardOffsetUnits=m  TranslationStandardAxis=+Z  TranslationCartesianOffset=[ankle_motor_offset_x -ankle_motor_offset_y ankle_motor_offset_z]  TranslationCartesianOffsetUnits=m  TranslationROffset=0  TranslationROffsetUnits=m  TranslationZOffset=0  TranslationZOffsetUnits=m  TranslationThetaOffset=0  TranslationThetaOffsetUnits=deg  RotationMethod=StandardAxis  RotationAngleUnits=deg  RotationStandardAxis=+Z  RotationAngle=180  RotationArbitraryAxis=[0 0 1]  FollAlignAxisA=+X  BaseAlignAxisA=+Y  FollAlignAxisB=+Y  BaseAlignAxisB=+Z  RotationSequenceAxes=FollowerAxes  RotationSequence=XYX  RotationSequenceAngles=[0 0 0]  RotationSequenceAnglesUnits=deg  RotationMatrix=[1 0 0; 0 1 0; 0 0 1]  Quaternion=[1 0 0 0]
  Rigid Transform2 : sm_lib/Frames and Transforms/Rigid Transform  TranslationMethod=None  TranslationStandardOffset=0.014  TranslationStandardOffsetUnits=m  TranslationStandardAxis=+Y  TranslationCartesianOffset=[0 0 0]  TranslationCartesianOffsetUnits=m  TranslationROffset=0  TranslationROffsetUnits=m  TranslationZOffset=0  TranslationZOffsetUnits=m  TranslationThetaOffset=0  TranslationThetaOffsetUnits=deg  RotationMethod=StandardAxis  RotationAngleUnits=deg  RotationStandardAxis=-X  RotationAngle=90  RotationArbitraryAxis=[0 0 1]  FollAlignAxisA=+X  BaseAlignAxisA=+Y  FollAlignAxisB=+Y  BaseAlignAxisB=+Z  RotationSequenceAxes=FollowerAxes  RotationSequence=XYX  RotationSequenceAngles=[0 0 0]  RotationSequenceAnglesUnits=deg  RotationMatrix=[1 0 0; 0 1 0; 0 0 1]  Quaternion=[1 0 0 0]
  Rigid Transform3 : sm_lib/Frames and Transforms/Rigid Transform  TranslationMethod=None  TranslationStandardOffset=0  TranslationStandardOffsetUnits=m  TranslationStandardAxis=+Z  TranslationCartesianOffset=[0 0 0]  TranslationCartesianOffsetUnits=m  TranslationROffset=0  TranslationROffsetUnits=m  TranslationZOffset=0  TranslationZOffsetUnits=m  TranslationThetaOffset=0  TranslationThetaOffsetUnits=deg  RotationMethod=StandardAxis  RotationAngleUnits=deg  RotationStandardAxis=+X  RotationAngle=90  RotationArbitraryAxis=[0 0 1]  FollAlignAxisA=+X  BaseAlignAxisA=+Y  FollAlignAxisB=+Y  BaseAlignAxisB=+Z  RotationSequenceAxes=FollowerAxes  RotationSequence=XYX  RotationSequenceAngles=[0 0 0]  RotationSequenceAnglesUnits=deg  RotationMatrix=[1 0 0; 0 1 0; 0 0 1]  Quaternion=[1 0 0 0]
  Rigid Transform4 : sm_lib/Frames and Transforms/Rigid Transform  TranslationMethod=Cartesian  TranslationStandardOffset=0  TranslationStandardOffsetUnits=m  TranslationStandardAxis=+Z  TranslationCartesianOffset=[knee_motor_offset_x -knee_motor_offset_y knee_motor_offset_z]  TranslationCartesianOffsetUnits=m  TranslationROffset=0  TranslationROffsetUnits=m  TranslationZOffset=0  TranslationZOffsetUnits=m  TranslationThetaOffset=0  TranslationThetaOffsetUnits=deg  RotationMethod=StandardAxis  RotationAngleUnits=deg  RotationStandardAxis=+Z  RotationAngle=180  RotationArbitraryAxis=[0 0 1]  FollAlignAxisA=+X  BaseAlignAxisA=+Y  FollAlignAxisB=+Y  BaseAlignAxisB=+Z  RotationSequenceAxes=FollowerAxes  RotationSequence=XYX  RotationSequenceAngles=[0 0 0]  RotationSequenceAnglesUnits=deg  RotationMatrix=[1 0 0; 0 1 0; 0 0 1]  Quaternion=[1 0 0 0]
  Thigh : sm_lib/Body Elements/File Solid  ExtGeomFileName=STL files\R_thigh.STL  UnitType=Custom  ExtGeomFileUnits=m  StepReaderType=HEX  ExportConvexHullGeometry=off  InertiaType=Custom  Mass=thigh_mass  MassUnits=kg  CenterOfMass=[thigh_com_x thigh_com_y thigh_com_z]  CenterOfMassUnits=m  MomentsOfInertia=[thigh_ixx thigh_iyy thigh_izz]  MomentsOfInertiaUnits=kg*m^2  ProductsOfInertia=[0 0 0]  ProductsOfInertiaUnits=kg*m^2  BasedOnType=Density  Density=1000  DensityUnits=kg/m^3  DoExposeReferenceFrame=on  SerializedFrames=<Frames/>  GraphicType=FromGeometry  MarkerShape=Sphere  MarkerSize=10  GraphicVisPropType=AdvancedVisualProperties  GraphicDiffuseColor=[0.9 0.9 0.9]  GraphicSpecularColor=[0.7 0.7 0.7 1.0]  GraphicAmbientColor=[0.35 0.35 0.35 1.0]  GraphicEmissiveColor=[0.0 0.0 0.0 1.0]  GraphicShininess=5  GraphicOpacity=1.0
  ankle motor : sm_lib/Body Elements/File Solid  ExtGeomFileName=STL files/A1motor_mirror.STL  UnitType=Custom  ExtGeomFileUnits=m  StepReaderType=HEX  ExportConvexHullGeometry=off  InertiaType=Custom  Mass=0.605  MassUnits=kg  CenterOfMass=motor_com_mirror  CenterOfMassUnits=m  MomentsOfInertia=motor_I  MomentsOfInertiaUnits=kg*m^2  ProductsOfInertia=[0 0 0]  ProductsOfInertiaUnits=kg*m^2  BasedOnType=DensityFromFile  Density=1000  DensityUnits=kg/m^3  DoExposeReferenceFrame=on  SerializedFrames=<Frames/>  GraphicType=None  MarkerShape=Sphere  MarkerSize=10  GraphicVisPropType=SimpleVisualProperties  GraphicDiffuseColor=[0.2 0.2 0.2]  GraphicSpecularColor=[0.5 0.5 0.5 1.0]  GraphicAmbientColor=[0.15 0.15 0.15 1.0]  GraphicEmissiveColor=[0.0 0.0 0.0 1.0]  GraphicShininess=75  GraphicOpacity=1.0
  knee motor : sm_lib/Body Elements/File Solid  ExtGeomFileName=STL files/A1motor_mirror.STL  UnitType=Custom  ExtGeomFileUnits=m  StepReaderType=HEX  ExportConvexHullGeometry=off  InertiaType=Custom  Mass=0.605  MassUnits=kg  CenterOfMass=motor_com_mirror  CenterOfMassUnits=m  MomentsOfInertia=motor_I  MomentsOfInertiaUnits=kg*m^2  ProductsOfInertia=[0 0 0]  ProductsOfInertiaUnits=kg*m^2  BasedOnType=DensityFromFile  Density=1000  DensityUnits=kg/m^3  DoExposeReferenceFrame=on  SerializedFrames=<Frames/>  GraphicType=None  MarkerShape=Sphere  MarkerSize=10  GraphicVisPropType=SimpleVisualProperties  GraphicDiffuseColor=[0.2 0.2 0.2]  GraphicSpecularColor=[0.5 0.5 0.5 1.0]  GraphicAmbientColor=[0.15 0.15 0.15 1.0]  GraphicEmissiveColor=[0.0 0.0 0.0 1.0]  GraphicShininess=75  GraphicOpacity=1.0
  B : PMIOPort  Side=Left
  ankle_motor : PMIOPort  Port=2  Side=Right
  F : PMIOPort  Port=3  Side=Right
  Sensor : Outport
  wires:
  Hip Pitch Joint/1(Sensor) -> Sensor/1
  Joint/1 -> Hip Pitch Joint/1(Joint)
  connections:
  Rigid Transform3/LConn1 -- Rigid Transform2/RConn1 -- Hip Pitch Joint/RConn1
  Hip Pitch Joint/LConn1 -- B/RConn1
  F/RConn1 -- Rigid Transform3/RConn1
  Thigh/RConn1 -- Rigid Transform1/LConn1 -- Rigid Transform4/LConn1 -- Rigid Transform2/LConn1
  ankle motor/RConn1 -- Rigid Transform1/RConn1 -- ankle_motor/RConn1
  knee motor/RConn1 -- Rigid Transform4/RConn1

== system Hector_Simulation/Hector/Right Leg/calf ==
  Joint : Inport
  Knee Joint : Subsystem
      settings: PortSchema="{\"entries\":[{\"content\":{\"sides\":[{\"content\":{\"connectorIds\":[\"LConn1\",\"In1\"]},\"type\":\"ConnectorPlacement.EquallySpacedRectSide\",\"uuid\":\"fe1bafd1-c1a5-4148-b465-5de294b235b8\"},{\"content\":{\"connectorIds\":[\"RConn1\",\"Out1\",\"Out2\",\"Out3\"],\"side\":\"RIGHT\"},\"type\":\"ConnectorPlacement.EquallySpacedRectSide\",\"uuid\":\"cbba8e06-0841-4611-b08d-047237296da9\"},{\"content\":{\"connectorIds\":[],\"side\":\"TOP\"},\"type\":\"ConnectorPlacement.EquallySpacedRectSide\",\"uuid\":\"b5035594-e8f7-4741-b410-9cfafd0751b0\"}]},\"type\":\"ConnectorPlacement.EquallySpacedConnector\",\"uuid\":\"2233606c-74e6-45bf-8a73-f401921fd730\"}],\"packageUris\":[\"http://schema.mathworks.com/mf0/Connector/R2020b\"],\"version\":\"1.0\"}"
  Rigid Transform4 : sm_lib/Frames and Transforms/Rigid Transform  TranslationMethod=None  TranslationStandardOffset=0  TranslationStandardOffsetUnits=m  TranslationStandardAxis=+Z  TranslationCartesianOffset=[0 0 0]  TranslationCartesianOffsetUnits=m  TranslationROffset=0  TranslationROffsetUnits=m  TranslationZOffset=0  TranslationZOffsetUnits=m  TranslationThetaOffset=0  TranslationThetaOffsetUnits=deg  RotationMethod=StandardAxis  RotationAngleUnits=deg  RotationStandardAxis=-X  RotationAngle=90  RotationArbitraryAxis=[0 0 1]  FollAlignAxisA=+X  BaseAlignAxisA=+Y  FollAlignAxisB=+Y  BaseAlignAxisB=+Z  RotationSequenceAxes=FollowerAxes  RotationSequence=XYX  RotationSequenceAngles=[0 0 0]  RotationSequenceAnglesUnits=deg  RotationMatrix=[1 0 0; 0 1 0; 0 0 1]  Quaternion=[1 0 0 0]
  Rigid Transform5 : sm_lib/Frames and Transforms/Rigid Transform  TranslationMethod=None  TranslationStandardOffset=0  TranslationStandardOffsetUnits=m  TranslationStandardAxis=+Z  TranslationCartesianOffset=[0 0 0]  TranslationCartesianOffsetUnits=m  TranslationROffset=0  TranslationROffsetUnits=m  TranslationZOffset=0  TranslationZOffsetUnits=m  TranslationThetaOffset=0  TranslationThetaOffsetUnits=deg  RotationMethod=StandardAxis  RotationAngleUnits=deg  RotationStandardAxis=+X  RotationAngle=90  RotationArbitraryAxis=[0 0 1]  FollAlignAxisA=+X  BaseAlignAxisA=+Y  FollAlignAxisB=+Y  BaseAlignAxisB=+Z  RotationSequenceAxes=FollowerAxes  RotationSequence=XYX  RotationSequenceAngles=[0 0 0]  RotationSequenceAnglesUnits=deg  RotationMatrix=[1 0 0; 0 1 0; 0 0 1]  Quaternion=[1 0 0 0]
  calf : sm_lib/Body Elements/File Solid  ExtGeomFileName=STL files\R_calf.STL  UnitType=Custom  ExtGeomFileUnits=m  StepReaderType=HEX  ExportConvexHullGeometry=off  InertiaType=Custom  Mass=calf_mass  MassUnits=kg  CenterOfMass=[calf_com_x calf_com_y calf_com_z]  CenterOfMassUnits=m  MomentsOfInertia=[calf_ixx calf_iyy calf_izz]  MomentsOfInertiaUnits=kg*m^2  ProductsOfInertia=[0 0 0]  ProductsOfInertiaUnits=kg*m^2  BasedOnType=Density  Density=1000  DensityUnits=kg/m^3  DoExposeReferenceFrame=on  SerializedFrames=<Frames/>  GraphicType=FromGeometry  MarkerShape=Sphere  MarkerSize=10  GraphicVisPropType=AdvancedVisualProperties  GraphicDiffuseColor=[0.9 0.9 0.9]  GraphicSpecularColor=[0.7 0.7 0.7 1.0]  GraphicAmbientColor=[0.35 0.35 0.35 1.0]  GraphicEmissiveColor=[0.0 0.0 0.0 1.0]  GraphicShininess=5  GraphicOpacity=1.0
  B : PMIOPort  Side=Left
  Conn2 : PMIOPort  Port=2  Side=Right
  Sensor : Outport
  knee_angle : Outport  Port=2
  knee_angle_speed : Outport  Port=3
  wires:
  Knee Joint/2(knee_angle) -> knee_angle/1
  Knee Joint/3(knee_angle_speed) -> knee_angle_speed/1
  Knee Joint/1(Sensor) -> Sensor/1
  Joint/1 -> Knee Joint/1(Joint)
  connections:
  calf/RConn1 -- Rigid Transform4/LConn1
  Knee Joint/LConn1 -- B/RConn1
  Rigid Transform5/LConn1 -- Knee Joint/RConn1 -- Rigid Transform4/RConn1
  Rigid Transform5/RConn1 -- Conn2/RConn1

== system Hector_Simulation/Hector/Right Leg/foot ==
  input : Inport
  Ankle Joint : Subsystem
      settings: PortSchema="{\"entries\":[{\"content\":{\"sides\":[{\"content\":{\"connectorIds\":[\"LConn1\",\"In1\"]},\"type\":\"ConnectorPlacement.EquallySpacedRectSide\",\"uuid\":\"d1094410-d7e2-420f-9299-c6db7682fd14\"},{\"content\":{\"connectorIds\":[\"RConn1\",\"Out1\"],\"side\":\"RIGHT\"},\"type\":\"ConnectorPlacement.EquallySpacedRectSide\",\"uuid\":\"17ca1f8d-2ad9-48dc-a054-4cdfe8b39b0e\"},{\"content\":{\"side\":\"TOP\"},\"type\":\"ConnectorPlacement.EquallySpacedRectSide\",\"uuid\":\"c0a1fb68-cc05-4666-9aff-395b76c49866\"}]},\"type\":\"ConnectorPlacement.EquallySpacedConnector\",\"uuid\":\"a0ca8f3e-9cc5-4e2d-aebb-075ea702600d\"}],\"packageUris\":[\"http://schema.mathworks.com/mf0/Connector/R2020b\"],\"version\":\"1.0\"}"
  Foot : sm_lib/Body Elements/File Solid  ExtGeomFileName=STL files\L_foot.STL  UnitType=Custom  ExtGeomFileUnits=m  StepReaderType=HEX  ExportConvexHullGeometry=off  InertiaType=Custom  Mass=toe_mass  MassUnits=kg  CenterOfMass=[toe_com_x -toe_com_y toe_com_z]  CenterOfMassUnits=m  MomentsOfInertia=[toe_ixx toe_iyy toe_izz]  MomentsOfInertiaUnits=kg*m^2  ProductsOfInertia=[0 0 0]  ProductsOfInertiaUnits=kg*m^2  BasedOnType=Density  Density=1000  DensityUnits=kg/m^3  DoExposeReferenceFrame=on  SerializedFrames=<Frames/>  GraphicType=FromGeometry  MarkerShape=Sphere  MarkerSize=10  GraphicVisPropType=AdvancedVisualProperties  GraphicDiffuseColor=[0.9 0.9 0.9]  GraphicSpecularColor=[0.7 0.7 0.7 1.0]  GraphicAmbientColor=[0.35 0.35 0.35 1.0]  GraphicEmissiveColor=[0.0 0.0 0.0 1.0]  GraphicShininess=5  GraphicOpacity=1.0
  Rigid Transform : sm_lib/Frames and Transforms/Rigid Transform  TranslationMethod=Cartesian  TranslationStandardOffset=0  TranslationStandardOffsetUnits=m  TranslationStandardAxis=+Z  TranslationCartesianOffset=[0 0.01 0]  TranslationCartesianOffsetUnits=m  TranslationROffset=0  TranslationROffsetUnits=m  TranslationZOffset=0  TranslationZOffsetUnits=m  TranslationThetaOffset=0  TranslationThetaOffsetUnits=deg  RotationMethod=None  RotationAngleUnits=deg  RotationStandardAxis=+Z  RotationAngle=0.0  RotationArbitraryAxis=[0 0 1]  FollAlignAxisA=+X  BaseAlignAxisA=+Y  FollAlignAxisB=+Y  BaseAlignAxisB=+Z  RotationSequenceAxes=FollowerAxes  RotationSequence=XYX  RotationSequenceAngles=[0 0 0]  RotationSequenceAnglesUnits=deg  RotationMatrix=[1 0 0; 0 1 0; 0 0 1]  Quaternion=[1 0 0 0]
  Rigid Transform6 : sm_lib/Frames and Transforms/Rigid Transform  TranslationMethod=None  TranslationStandardOffset=0  TranslationStandardOffsetUnits=m  TranslationStandardAxis=+Z  TranslationCartesianOffset=[0 0 0]  TranslationCartesianOffsetUnits=m  TranslationROffset=0  TranslationROffsetUnits=m  TranslationZOffset=0  TranslationZOffsetUnits=m  TranslationThetaOffset=0  TranslationThetaOffsetUnits=deg  RotationMethod=StandardAxis  RotationAngleUnits=deg  RotationStandardAxis=-X  RotationAngle=90  RotationArbitraryAxis=[0 0 1]  FollAlignAxisA=+X  BaseAlignAxisA=+Y  FollAlignAxisB=+Y  BaseAlignAxisB=+Z  RotationSequenceAxes=FollowerAxes  RotationSequence=XYX  RotationSequenceAngles=[0 0 0]  RotationSequenceAnglesUnits=deg  RotationMatrix=[1 0 0; 0 1 0; 0 0 1]  Quaternion=[1 0 0 0]
  B : PMIOPort  Side=Left
  Conn4 : PMIOPort  Port=2  Side=Right
  F : PMIOPort  Port=3  Side=Right
  sensor : Outport
  wires:
  input/1 -> Ankle Joint/1(input)
  Ankle Joint/1(sensor) -> sensor/1
  connections:
  Rigid Transform6/RConn1 -- Ankle Joint/RConn1
  Ankle Joint/LConn1 -- B/RConn1
  Rigid Transform/RConn1 -- Conn4/RConn1 -- Rigid Transform6/LConn1 -- F/RConn1
  Rigid Transform/LConn1 -- Foot/RConn1
